simulink model "PositionControlPtos"  (R2020a)
settings: Solver=ode3  StartTime=0.0  StopTime=100.0  FixedStep=Ts  RelTol=1e-3
values from neighbouring files (symbols this model uses):
  obsx = 1.5    [RunEvitarObstaculo.m]    (also in runPositionControlTray.m = 4)
  obsy = 1    [RunEvitarObstaculo.m]    (also in runPositionControlTray.m = 0.5)
  refx = 5    [RunEvitarObstaculo.m]
  refy = 5    [RunEvitarObstaculo.m]
undefined symbols (not defined in the file or in its folder): DiscIntNeverNeededParam
libraries: fuzblock x1, simulink x1
settings Model: Creator=pizarro  LastModifiedBy=Javier
settings DataIOCC: ReturnWorkspaceOutputs=off
settings SFSimCC: CustomCodeUndefinedFunction=UseInterfaceOnly

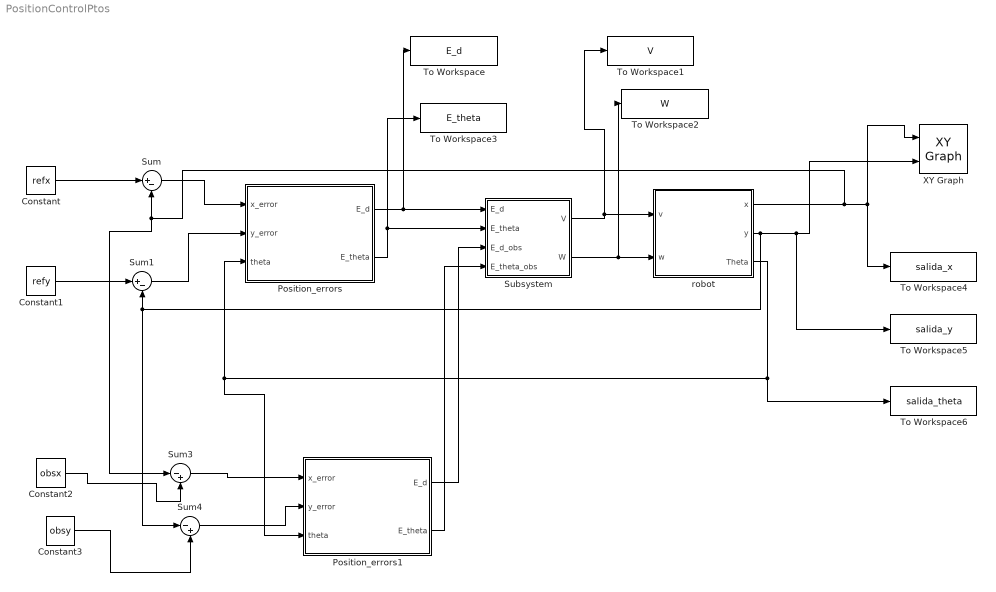
== system PositionControlPtos ==
  Constant : Constant  Value=refx
  Constant1 : Constant  Value=refy
  Constant2 : Constant  Value=obsx
  Constant3 : Constant  Value=obsy
  Position_errors : Subsystem
  Position_errors1 : Subsystem
  Subsystem : Subsystem
  Sum : Sum  Inputs=|+-
  Sum1 : Sum  Inputs=|+-
  Sum3 : Sum  Inputs=|-+
  Sum4 : Sum  Inputs=|-+
  To Workspace : ToWorkspace  VariableName=E_d  SaveFormat=Structure With Time  SampleTime=-1
  To Workspace1 : ToWorkspace  VariableName=V  SaveFormat=Structure With Time  SampleTime=-1
  To Workspace2 : ToWorkspace  VariableName=W  SaveFormat=Structure With Time  SampleTime=-1
  To Workspace3 : ToWorkspace  VariableName=E_theta  SaveFormat=Structure With Time  SampleTime=-1
  To Workspace4 : ToWorkspace  VariableName=salida_x  SaveFormat=Structure With Time  SampleTime=-1
  To Workspace5 : ToWorkspace  VariableName=salida_y  SaveFormat=Structure With Time  SampleTime=-1
  To Workspace6 : ToWorkspace  VariableName=salida_theta  SaveFormat=Structure With Time  SampleTime=-1
  XY Graph : simulink/Sinks/XY Graph  xmin=-5  xmax=100  ymin=-5  ymax=100  st=-1
  robot : Subsystem
  wires:
  Position_errors/1(E_d) -> Subsystem/1(E_d), To Workspace/1
  Position_errors/2(E_theta) -> Subsystem/2(E_theta), To Workspace3/1
  Subsystem/1(V) -> To Workspace1/1, robot/1(v)
  Subsystem/2(W) -> To Workspace2/1, robot/2(w)
  Sum/1 -> Position_errors/1(x_error)
  Sum1/1 -> Position_errors/2(y_error)
  robot/1(x) -> Sum3/1, Sum/2, XY Graph/1, To Workspace4/1
  robot/2(y) -> To Workspace5/1, XY Graph/2, Sum4/1, Sum1/2
  robot/3(Theta) -> Position_errors1/3(theta), Position_errors/3(theta), To Workspace6/1
  Constant/1 -> Sum/1
  Constant1/1 -> Sum1/1
  Constant2/1 -> Sum3/2
  Constant3/1 -> Sum4/2
  Sum3/1 -> Position_errors1/1(x_error)
  Sum4/1 -> Position_errors1/2(y_error)
  Position_errors1/1(E_d) -> Subsystem/3(E_d_obs)
  Position_errors1/2(E_theta) -> Subsystem/4(E_theta_obs)

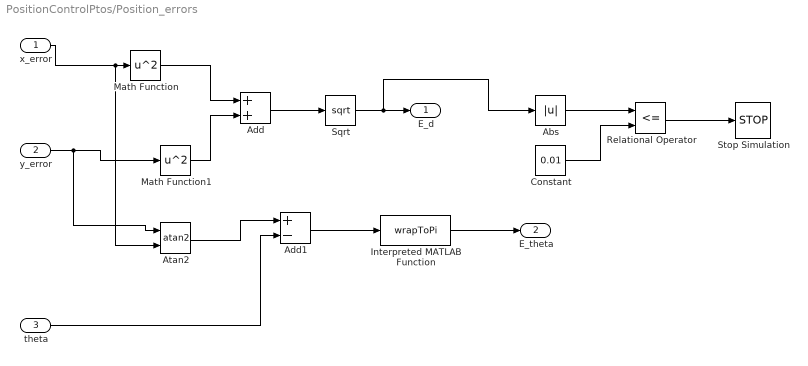
== system PositionControlPtos/Position_errors ==
  x_error : Inport
  y_error : Inport  Port=2
  theta : Inport  Port=3
  Abs : Abs
  Add : Sum
  Add1 : Sum  Inputs=+-
  Atan2 : Trigonometry  Operator=atan2  OutputSignalType=real
  Constant : Constant  Value=0.01
  Interpreted MATLAB Function : MATLABFcn  MATLABFcn=wrapToPi
  Math Function : Math  Operator=square  SaturateOnIntegerOverflow=on
  Math Function1 : Math  Operator=square  SaturateOnIntegerOverflow=on
  Relational Operator : RelationalOperator  Operator=<=  OutDataTypeStr=boolean  RndMeth=Simplest
  Sqrt : Sqrt  SaturateOnIntegerOverflow=on
  Stop Simulation : Stop
  E_d : Outport
  E_theta : Outport  Port=2
  wires:
  x_error/1 -> Atan2/2, Math Function/1
  y_error/1 -> Atan2/1, Math Function1/1
  Math Function/1 -> Add/1
  Math Function1/1 -> Add/2
  Add/1 -> Sqrt/1
  Sqrt/1 -> Abs/1, E_d/1
  Atan2/1 -> Add1/1
  theta/1 -> Add1/2
  Abs/1 -> Relational Operator/1
  Constant/1 -> Relational Operator/2
  Relational Operator/1 -> Stop Simulation/1
  Add1/1 -> Interpreted MATLAB Function/1
  Interpreted MATLAB Function/1 -> E_theta/1

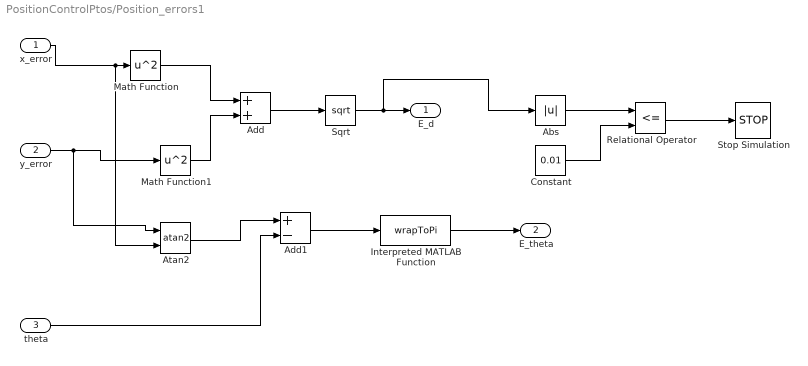
== system PositionControlPtos/Position_errors1 ==
  x_error : Inport
  y_error : Inport  Port=2
  theta : Inport  Port=3
  Abs : Abs
  Add : Sum
  Add1 : Sum  Inputs=+-
  Atan2 : Trigonometry  Operator=atan2  OutputSignalType=real
  Constant : Constant  Value=0.01
  Interpreted MATLAB Function : MATLABFcn  MATLABFcn=wrapToPi
  Math Function : Math  Operator=square  SaturateOnIntegerOverflow=on
  Math Function1 : Math  Operator=square  SaturateOnIntegerOverflow=on
  Relational Operator : RelationalOperator  Operator=<=  OutDataTypeStr=boolean  RndMeth=Simplest
  Sqrt : Sqrt  SaturateOnIntegerOverflow=on
  Stop Simulation : Stop
  E_d : Outport
  E_theta : Outport  Port=2
  wires:
  x_error/1 -> Atan2/2, Math Function/1
  y_error/1 -> Atan2/1, Math Function1/1
  Math Function/1 -> Add/1
  Math Function1/1 -> Add/2
  Add/1 -> Sqrt/1
  Sqrt/1 -> Abs/1, E_d/1
  Atan2/1 -> Add1/1
  theta/1 -> Add1/2
  Abs/1 -> Relational Operator/1
  Constant/1 -> Relational Operator/2
  Relational Operator/1 -> Stop Simulation/1
  Add1/1 -> Interpreted MATLAB Function/1
  Interpreted MATLAB Function/1 -> E_theta/1

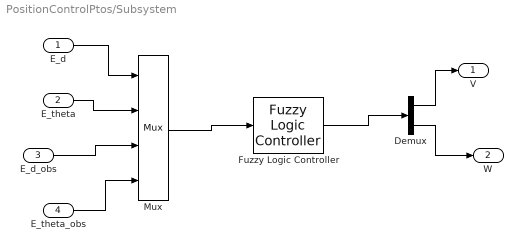
== system PositionControlPtos/Subsystem ==
  E_d : Inport
  E_theta : Inport  Port=2
  E_d_obs : Inport  Port=3
  E_theta_obs : Inport  Port=4
  Demux : Demux  Outputs=2
  Fuzzy Logic Controller : fuzblock/Fuzzy Logic  Controller  FIS='controlador.fis'  OutputSampleNumber=101  DataType=double  FuzzifiedInputs=off  RuleFiringStrengths=off  RuleOutputs=off  AggregatedOutputs=off  SimulateUsing=Interpreted execution  OutOfRangeInputValueMessage=warning  NoRuleFiredMessage=warning  EmptyOutputFuzzySetMessage=warning
  Mux : Mux
  V : Outport
  W : Outport  Port=2
  wires:
  Mux/1 -> Fuzzy Logic Controller/1
  Fuzzy Logic Controller/1 -> Demux/1
  E_d/1 -> Mux/1
  E_theta/1 -> Mux/2
  Demux/1 -> V/1
  Demux/2 -> W/1
  E_d_obs/1 -> Mux/3
  E_theta_obs/1 -> Mux/4

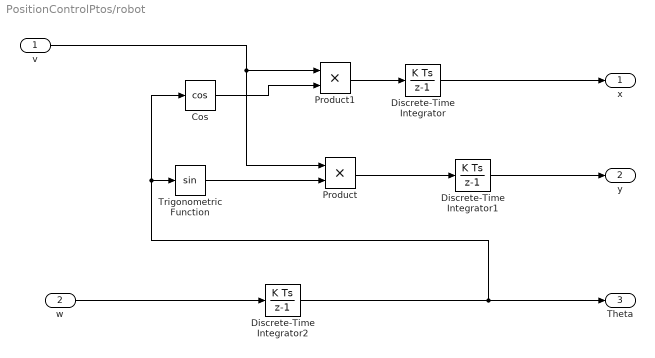
== system PositionControlPtos/robot ==
  v : Inport
  w : Inport  Port=2
  Cos : Trigonometry  Operator=cos
  Discrete-Time Integrator : DiscreteIntegrator  SampleTime=-1  ICPrevOutput=DiscIntNeverNeededParam  ICPrevScaledInput=DiscIntNeverNeededParam
  Discrete-Time Integrator1 : DiscreteIntegrator  SampleTime=-1  ICPrevOutput=DiscIntNeverNeededParam  ICPrevScaledInput=DiscIntNeverNeededParam
  Discrete-Time Integrator2 : DiscreteIntegrator  SampleTime=-1  ICPrevOutput=DiscIntNeverNeededParam  ICPrevScaledInput=DiscIntNeverNeededParam
  Product : Product
  Product1 : Product
  Trigonometric Function : Trigonometry
  x : Outport
  y : Outport  Port=2
  Theta : Outport  Port=3
  wires:
  Trigonometric Function/1 -> Product/2
  Discrete-Time Integrator/1 -> x/1
  Cos/1 -> Product1/2
  Product/1 -> Discrete-Time Integrator1/1
  Discrete-Time Integrator2/1 -> Theta/1, Cos/1, Trigonometric Function/1
  Product1/1 -> Discrete-Time Integrator/1
  Discrete-Time Integrator1/1 -> y/1
  w/1 -> Discrete-Time Integrator2/1
  v/1 -> Product/1, Product1/1
